simulink model "inverse_funtion"  (R2024b)
settings: Solver=VariableStepAuto  StartTime=0.0  StopTime=5  RelTol=1e-3
settings Model: Creator=Lenovo  LastModifiedBy=Lenovo

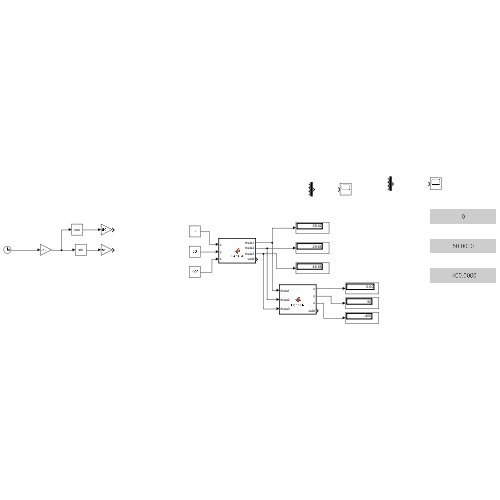
[thumbnail: Simulink's stored preview of the top-level diagram]
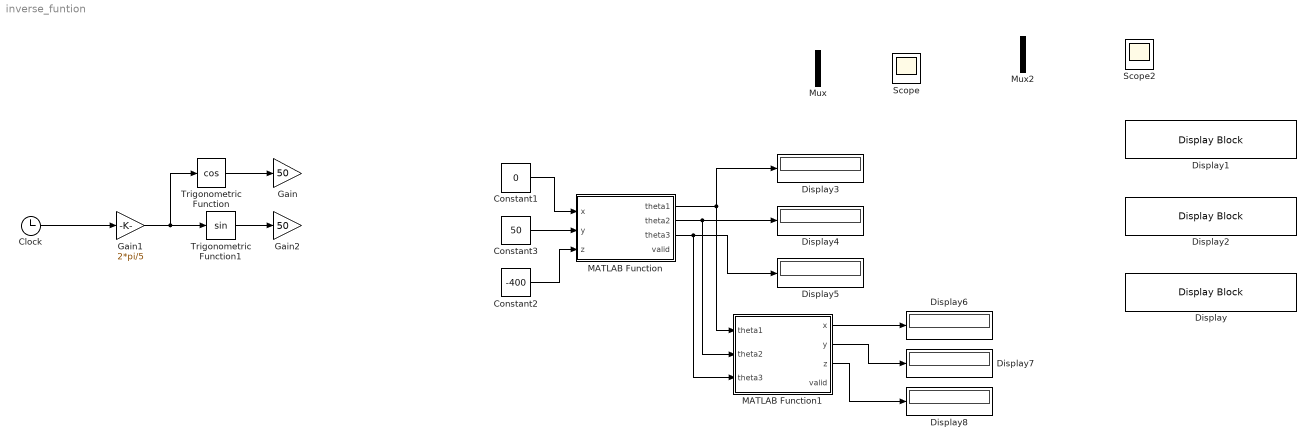
== system inverse_funtion ==
  Clock : Clock
  Constant1 : Constant  Value=0
  Constant2 : Constant  Value=-400
  Constant3 : Constant  Value=50
  Display : DisplayBlock  LabelPosition=Hide  Transparency=1
  Display1 : DisplayBlock  LabelPosition=Hide  Format=Integer  Transparency=1
  Display2 : DisplayBlock  LabelPosition=Hide  Transparency=1
  Display{3..8} (6 alike) : Display
      Display6 settings: Format=bank
  Gain : Gain  Gain=50
  Gain1 : Gain  Gain=2*pi/5
  Gain2 : Gain  Gain=50
  MATLAB Function : MATLAB Function  TreatAsAtomicUnit=on
  MATLAB Function1 : MATLAB Function  TreatAsAtomicUnit=on
  Mux : Mux  Inputs=3
  Mux2 : Mux  Inputs=3
  Scope : Scope
  Scope2 : Scope
  Trigonometric Function : Trigonometry  Operator=cos
  Trigonometric Function1 : Trigonometry
  wires:
  Constant2/1 -> MATLAB Function/3(z)
  MATLAB Function/1(theta1) -> Display3/1, MATLAB Function1/1(theta1)
  Trigonometric Function/1 -> Gain/1
  Clock/1 -> Gain1/1
  Trigonometric Function1/1 -> Gain2/1
  Gain1/1 -> Trigonometric Function/1, Trigonometric Function1/1
  MATLAB Function/2(theta2) -> Display4/1, MATLAB Function1/2(theta2)
  MATLAB Function/3(theta3) -> Display5/1, MATLAB Function1/3(theta3)
  Constant3/1 -> MATLAB Function/2(y)
  Constant1/1 -> MATLAB Function/1(x)
  MATLAB Function1/1(x) -> Display6/1
  MATLAB Function1/2(y) -> Display7/1
  MATLAB Function1/3(z) -> Display8/1

== matlab function inverse_funtion/MATLAB Function1 ==
  data: x output; theta1 input; y output; theta2 input; theta3 input; z output; valid output
function [x, y, z, valid] = DeltaFK(theta1, theta2, theta3)
%#codegen
% Delta机器人正运动学
%
% 输入：
% theta1,theta2,theta3   主动关节角 [deg]
%
% 输出：
% x,y,z                  动平台中心位置 [mm]
% valid                  1 = 正解有效
%                        0 = 当前角度无有效解

% --------------------------------
% 机器人参数
% --------------------------------
L1 = 200.0;
L2 = 380.0;

R = 180.0;
r = 80.0;

% 三个支链方位角
phi1 = 0.0;
phi2 = 2*pi/3;
phi3 = 4*pi/3;

% --------------------------------
% deg -> rad
% --------------------------------
t1 = theta1*pi/180;
t2 = theta2*pi/180;
t3 = theta3*pi/180;

% --------------------------------
% 计算三个等效球心
%
% 实际主动臂末端为 B_i
% 因为动平台铰点相对中心有 r 的偏移，
% 将球心平移 -r*u_i 后，
% 就可以直接求平台中心 P
% --------------------------------

d = R-r;

% 第一支链
Q1x = d*cos(phi1) + L1*cos(t1)*cos(phi1);
Q1y = d*sin(phi1) + L1*cos(t1)*sin(phi1);
Q1z = -L1*sin(t1);

% 第二支链
Q2x = d*cos(phi2) + L1*cos(t2)*cos(phi2);
Q2y = d*sin(phi2) + L1*cos(t2)*sin(phi2);
Q2z = -L1*sin(t2);

% 第三支链
Q3x = d*cos(phi3) + L1*cos(t3)*cos(phi3);
Q3y = d*sin(phi3) + L1*cos(t3)*sin(phi3);
Q3z = -L1*sin(t3);

% --------------------------------
% 建立两个平面方程
%
% |P-Q1|^2 = L2^2
% |P-Q2|^2 = L2^2
% |P-Q3|^2 = L2^2
%
% 球面方程相减后：
%
% A*x + B*y + C*z = D
% --------------------------------

A1 = 2*(Q2x-Q1x);
B1 = 2*(Q2y-Q1y);
C1 = 2*(Q2z-Q1z);

D1 = Q2x^2 + Q2y^2 + Q2z^2 ...
   - Q1x^2 - Q1y^2 - Q1z^2;

A2 = 2*(Q3x-Q1x);
B2 = 2*(Q3y-Q1y);
C2 = 2*(Q3z-Q1z);

D2 = Q3x^2 + Q3y^2 + Q3z^2 ...
   - Q1x^2 - Q1y^2 - Q1z^2;

% --------------------------------
% 两个平面的交线
%
% P = P0 + lambda*v
%
% v 为两个平面法向量叉乘
% --------------------------------

n1x = A1;
n1y = B1;
n1z = C1;

n2x = A2;
n2y = B2;
n2z = C2;

% v = n1 x n2
vx = n1y*n2z - n1z*n2y;
vy = n1z*n2x - n1x*n2z;
vz = n1x*n2y - n1y*n2x;

v2 = vx^2 + vy^2 + vz^2;

% 默认输出
x = 0.0;
y = 0.0;
z = 0.0;
valid = 0.0;

% 奇异情况保护
if v2 < 1e-12
    return;
end

% --------------------------------
% 求交线上的一个点 P0
%
% P0 = [D1*(n2 x v) + D2*(v x n1)] / |v|^2
% --------------------------------

% n2 x v
c1x = n2y*vz - n2z*vy;
c1y = n2z*vx - n2x*vz;
c1z = n2x*vy - n2y*vx;

% v x n1
c2x = vy*n1z - vz*n1y;
c2y = vz*n1x - vx*n1z;
c2z = vx*n1y - vy*n1x;

P0x = (D1*c1x + D2*c2x)/v2;
P0y = (D1*c1y + D2*c2y)/v2;
P0z = (D1*c1z + D2*c2z)/v2;

% --------------------------------
% 将交线代入第一个球面
%
% |P0 + lambda*v - Q1|^2 = L2^2
%
% 得到关于 lambda 的二次方程
% --------------------------------

wx = P0x-Q1x;
wy = P0y-Q1y;
wz = P0z-Q1z;

qa = v2;

qb = 2*(wx*vx + wy*vy + wz*vz);

qc = wx^2 + wy^2 + wz^2 - L2^2;

disc = qb^2 - 4*qa*qc;

% 没有实数交点
if disc < 0
    return;
end

sqrtDisc = sqrt(disc);

lambda1 = (-qb + sqrtDisc)/(2*qa);
lambda2 = (-qb - sqrtDisc)/(2*qa);

% 两个可能的空间交点
x1 = P0x + lambda1*vx;
y1 = P0y + lambda1*vy;
z1 = P0z + lambda1*vz;

x2 = P0x + lambda2*vx;
y2 = P0y + lambda2*vy;
z2 = P0z + lambda2*vz;

% --------------------------------
% Delta正常工作区域在固定平台下方
% 因此选择 z 更小的解
% --------------------------------

if z1 < z2
    x = x1;
    y = y1;
    z = z1;
else
    x = x2;
    y = y2;
    z = z2;
end

valid = 1.0;

end

== matlab function inverse_funtion/MATLAB Function ==
  data: x input; y input; theta1 output; z input; theta2 output; theta3 output; valid output
function [theta1, theta2, theta3, valid] = DeltaIK(x,y,z)
%#codegen
% =========================================================
% Delta机器人逆运动学
%
% 输入:
%   x,y,z       动平台中心位置 [mm]
%
% 输出:
%   theta1~3    三个主动关节角 [deg]
%   valid       1 = 有效
%               0 = 不可达
%
% 几何参数:
%   L1 = 200 mm
%   L2 = 380 mm
%   R  = 180 mm
%   r  = 80 mm
%
% 坐标定义:
%   z < 0       工作空间位于固定平台下方
%
% 角度定义:
%   theta = 0   主动臂水平向外
%   theta > 0   主动臂向下
% =========================================================


%% 机器人参数

L1 = 200.0;
L2 = 380.0;

R = 180.0;
r = 80.0;

d = R-r;


%% 三个支链方位角

phi1 = 0.0;

phi2 = 2.0*pi/3.0;

phi3 = 4.0*pi/3.0;


%% 分别计算三个关节角

[theta1,v1] = calcTheta(x,y,z,phi1,L1,L2,d);

[theta2,v2] = calcTheta(x,y,z,phi2,L1,L2,d);

[theta3,v3] = calcTheta(x,y,z,phi3,L1,L2,d);


%% 总体有效性

if (v1 > 0.5) && (v2 > 0.5) && (v3 > 0.5)

    valid = 1.0;

else

    valid = 0.0;

end

end



% =========================================================
% 单支链逆运动学
% =========================================================

function [theta,valid] = calcTheta(x,y,z,phi,L1,L2,d)

theta = 0.0;
valid = 0.0;


%% ---------------------------------------------------------
% 1. 将末端坐标转换到当前支链局部坐标
% ----------------------------------------------------------

% 径向分量
q = x*cos(phi) + y*sin(phi);

% 切向分量
s = -x*sin(phi) + y*cos(phi);


%% ---------------------------------------------------------
% 2. 固定平台与动平台铰点的径向差
% ----------------------------------------------------------

a = q-d;


%% ---------------------------------------------------------
% 3. 根据从动臂长度约束
%
% (a-L1*cos(theta))^2
% + s^2
% + (z+L1*sin(theta))^2
% = L2^2
%
% 展开得到：
%
% a*cos(theta) - z*sin(theta) = K
% ----------------------------------------------------------

K = (a*a + s*s + z*z + L1*L1 - L2*L2) ...
    /(2.0*L1);


%% ---------------------------------------------------------
% 4. 转换为标准三角方程
%
% a*cos(theta) - z*sin(theta) = K
%
% 定义：
%
% rho = sqrt(a^2+z^2)
%
% delta = atan2(-z,a)
%
% 则：
%
% rho*cos(theta-delta)=K
% ----------------------------------------------------------

rho = sqrt(a*a + z*z);

if rho < 1.0e-12
    return;
end

c = K/rho;


%% ---------------------------------------------------------
% 5. 工作空间检查
% ----------------------------------------------------------

tol = 1.0e-10;

if c > 1.0+tol
    return;
end

if c < -1.0-tol
    return;
end


% 防止浮点误差

if c > 1.0
    c = 1.0;
elseif c < -1.0
    c = -1.0;
end


%% ---------------------------------------------------------
% 6. 两个数学解
% ----------------------------------------------------------

delta = atan2(-z,a);

gamma = acos(c);


th1 = delta + gamma;

th2 = delta - gamma;


%% ---------------------------------------------------------
% 7. 归一化到 [-pi,pi]
% ----------------------------------------------------------

th1 = atan2(sin(th1),cos(th1));

th2 = atan2(sin(th2),cos(th2));


%% ---------------------------------------------------------
% 8. 选择正常Delta装配构型
%
% 当前假设机械关节范围：
%
% 0 <= theta <= 90 deg
% ----------------------------------------------------------

thetaMin = 0.0;

thetaMax = pi/2.0;


valid1 = (th1 >= thetaMin) && ...
         (th1 <= thetaMax);

valid2 = (th2 >= thetaMin) && ...
         (th2 <= thetaMax);


%% ---------------------------------------------------------
% 9. 选择物理解
% ----------------------------------------------------------

if valid1 && ~valid2

    thetaRad = th1;

elseif valid2 && ~valid1

    thetaRad = th2;

elseif valid1 && valid2

    % 两个都满足时选择较小角度
    if abs(th1) <= abs(th2)

        thetaRad = th1;

    else

        thetaRad = th2;

    end

else

    return;

end


%% ---------------------------------------------------------
% 10. 转换成 degree
% ----------------------------------------------------------

theta = thetaRad*180.0/pi;

valid = 1.0;

end
